simulink model "PassiveBalancingModelling"  (R2024b)
settings: Solver=FixedStepAuto  StartTime=0.0  StopTime=200  FixedStep=1e-3  RelTol=1e-3
model workspace (MAT data in the model file):
  Ah = 3
  R = 0.1
  SoC1 = 60
  SoC2 = 70
  SoC3 = 50
  SoC4 = 80
  Vnom = 3.7
undefined symbols (not defined in the file): Ion, Lithium
libraries: spsBatteryLib x4, spsIdealSwitchLib x4, spsSeriesRLCBranchLib x4, sps_lib x1
settings Model: Creator=MOHAMED  LastModifiedBy=MOHAMED

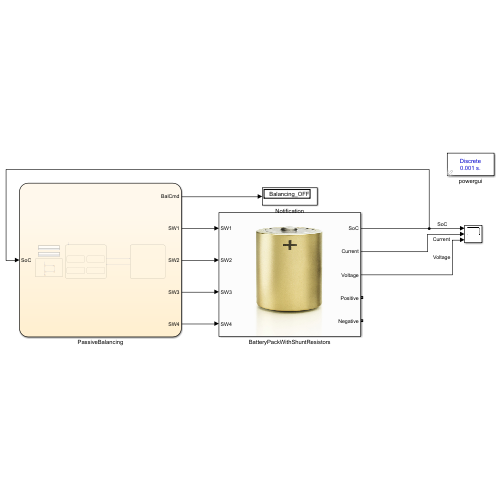
[thumbnail: Simulink's stored preview of the top-level diagram]
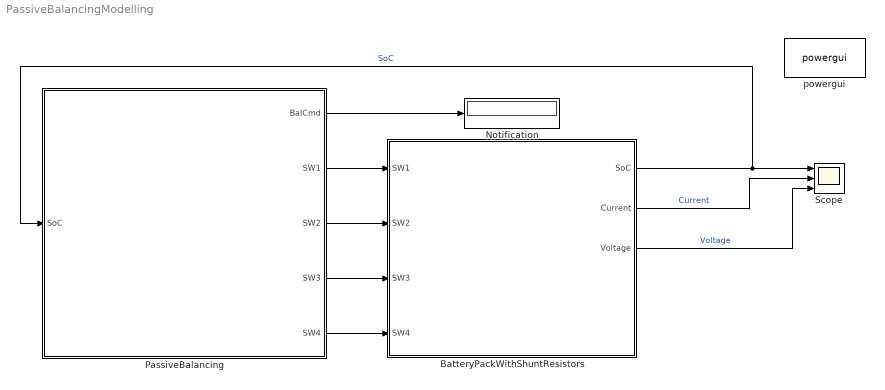
== system PassiveBalancingModelling ==
  BatteryPackWithShuntResistors : Subsystem
      mask Display: image('battery.jpg');
  Notification : Display
  PassiveBalancing : Stateflow chart  TreatAsAtomicUnit=on
  Scope : Scope  NumInputPorts=3
  powergui : sps_lib/powergui  Priority=1  SimulationMode=Discrete  SampleTime=1e-3  frequency=60  Iterations=50  frequencyindice=0  Pbase=100e6  ErrMax=1e-4  UnitsV=kV  UnitsW=MW  buscounter=0  FunctionMessages=off  echomessages=off  EnableUseOfTLC=off  CurrentSourceSwitches=off  DisableSnubberDevices=off  DisableRonSwitches=off  DisableVfSwitches=off  DisplayEquations=off  AutomaticDiscreteSolvers=off  SolverType=Tustin/Backward Euler (TBE)  Interpol=off  ExternalGateDelay=off  methode=off  Ts=100  x0status=blocks  SPID=on  SwTol=0  HookPort=off  NonlinearTolerance=1e-4  nMaxIteration=100  ContinueOnMaxIteration=off  RestoreLinks=warning  ResistiveCurrentMeasurement=off  Frange=[0:2:500]  Ylog=off  Xlog=on  ShowGrid=off  save=off  variable=ZData  structure=0  ZoomFFT=off  StartTime=0.0  cycles=1  DisplayStyle=1  fundamental=60  FreqAxis=off  MaxFrequency=1000  frequencyindicesteady=1  RmsSteady=1  display=off
  wires:
  BatteryPackWithShuntResistors/1(SoC) -> PassiveBalancing/1(SoC), Scope/1  "SoC"
  BatteryPackWithShuntResistors/2(Current) -> Scope/2  "Current"
  BatteryPackWithShuntResistors/3(Voltage) -> Scope/3  "Voltage"
  PassiveBalancing/1(BalCmd) -> Notification/1
  PassiveBalancing/2(SW1) -> BatteryPackWithShuntResistors/1(SW1)
  PassiveBalancing/3(SW2) -> BatteryPackWithShuntResistors/2(SW2)
  PassiveBalancing/4(SW3) -> BatteryPackWithShuntResistors/3(SW3)
  PassiveBalancing/5(SW4) -> BatteryPackWithShuntResistors/4(SW4)

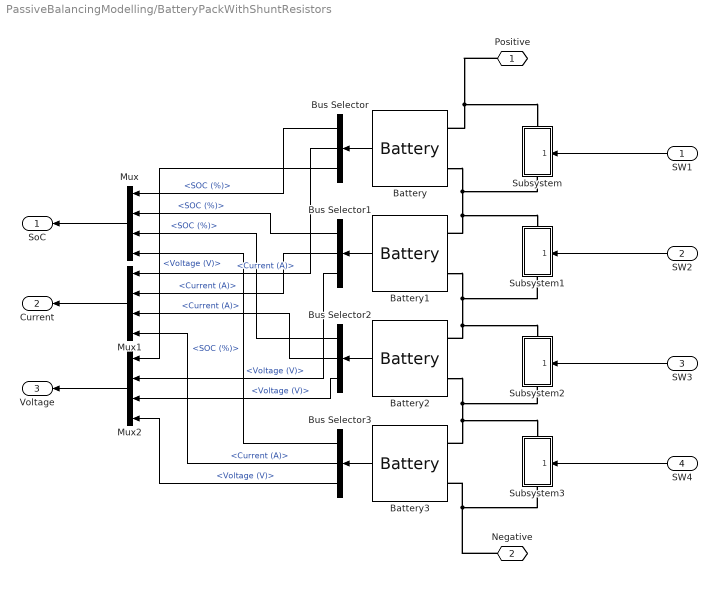
== system PassiveBalancingModelling/BatteryPackWithShuntResistors ==
  SW1 : Inport
  SW2 : Inport  Port=2
  SW3 : Inport  Port=3
  SW4 : Inport  Port=4
  Battery : spsBatteryLib/Battery  BatType=Lithium-Ion  NomV=Vnom  NomQ=Ah  SOC=SoC1  Batt_Tr=20e-3  PresetModel=on  MaxQ=3  MinV=2.775  FullV=4.3068  Dis_rate=1.3043  R=0.012333  Normal_OP=2.713  expZone="[3.9974     0.14739]"
  Battery1 : spsBatteryLib/Battery  BatType=Lithium-Ion  NomV=Vnom  NomQ=Ah  SOC=SoC2  Batt_Tr=20e-3  PresetModel=on  MaxQ=3  MinV=2.775  FullV=4.3068  Dis_rate=1.3043  R=0.012333  Normal_OP=2.713  expZone="[3.9974     0.14739]"
  Battery2 : spsBatteryLib/Battery  BatType=Lithium-Ion  NomV=Vnom  NomQ=Ah  SOC=SoC3  Batt_Tr=20e-3  PresetModel=on  MaxQ=3  MinV=2.775  FullV=4.3068  Dis_rate=1.3043  R=0.012333  Normal_OP=2.713  expZone="[3.9974     0.14739]"
  Battery3 : spsBatteryLib/Battery  BatType=Lithium-Ion  NomV=Vnom  NomQ=Ah  SOC=SoC4  Batt_Tr=20e-3  PresetModel=on  MaxQ=3  MinV=2.775  FullV=4.3068  Dis_rate=1.3043  R=0.012333  Normal_OP=2.713  expZone="[3.9974     0.14739]"
  Bus Selector{,1..3} (4 alike) : BusSelector  OutputSignals=SOC (%),Current (A),Voltage (V)
  Mux : Mux
  Mux1 : Mux
  Mux2 : Mux
  Subsystem : Subsystem
      settings: PortSchema="{\"entries\":[{\"content\":{\"sides\":[{\"content\":{\"connectorIds\":[\"LConn1\"]},\"type\":\"ConnectorPlacement.EquallySpacedRectSide\",\"uuid\":\"257d9981-230f-4391-a2c1-b56ae4b7ce10\"},{\"content\":{\"connectorIds\":[\"RConn1\"],\"side\":\"RIGHT\"},\"type\":\"ConnectorPlacement.EquallySpacedRectSide\",\"uuid\":\"90dd2fe2-2012-4c72-baa4-e13b85a759c3\"},{\"content\":{\"side\":\"TOP\"},\"type\":\"ConnectorPlacement.EquallySpacedRectSide\",\"uuid\":\"f37524ef-904f-4ff0-92c1-10d0565a33a2\"},{\"content\":{\"connectorIds\":[\"In1\"],\"side\":\"BOTTOM\"},\"type\":\"ConnectorPlacement.EquallySpacedRectSide\",\"uuid\":\"9c9ec85f-2592-4e7a-a4ab-a97d1a48809e\"}]},\"type\":\"ConnectorPlacement.EquallySpacedConnector\",\"uuid\":\"5659d0fe-4d8b-46d1-9b44-b48eced08a2e\"}],\"packageUris\":[\"http://schema.mathworks.com/mf0/Connector/R2020b\"],\"version\":\"1.0\"}"
  Subsystem1 : Subsystem
      settings: PortSchema="{\"entries\":[{\"content\":{\"sides\":[{\"content\":{\"connectorIds\":[\"LConn1\"]},\"type\":\"ConnectorPlacement.EquallySpacedRectSide\",\"uuid\":\"257d9981-230f-4391-a2c1-b56ae4b7ce10\"},{\"content\":{\"connectorIds\":[\"RConn1\"],\"side\":\"RIGHT\"},\"type\":\"ConnectorPlacement.EquallySpacedRectSide\",\"uuid\":\"90dd2fe2-2012-4c72-baa4-e13b85a759c3\"},{\"content\":{\"side\":\"TOP\"},\"type\":\"ConnectorPlacement.EquallySpacedRectSide\",\"uuid\":\"f37524ef-904f-4ff0-92c1-10d0565a33a2\"},{\"content\":{\"connectorIds\":[\"In1\"],\"side\":\"BOTTOM\"},\"type\":\"ConnectorPlacement.EquallySpacedRectSide\",\"uuid\":\"98333fe3-4431-4c4d-b596-c8152de66e7e\"}]},\"type\":\"ConnectorPlacement.EquallySpacedConnector\",\"uuid\":\"5659d0fe-4d8b-46d1-9b44-b48eced08a2e\"}],\"packageUris\":[\"http://schema.mathworks.com/mf0/Connector/R2020b\"],\"version\":\"1.0\"}"
  Subsystem2 : Subsystem
      settings: PortSchema="{\"entries\":[{\"content\":{\"sides\":[{\"content\":{\"connectorIds\":[\"LConn1\"]},\"type\":\"ConnectorPlacement.EquallySpacedRectSide\",\"uuid\":\"257d9981-230f-4391-a2c1-b56ae4b7ce10\"},{\"content\":{\"connectorIds\":[\"RConn1\"],\"side\":\"RIGHT\"},\"type\":\"ConnectorPlacement.EquallySpacedRectSide\",\"uuid\":\"90dd2fe2-2012-4c72-baa4-e13b85a759c3\"},{\"content\":{\"side\":\"TOP\"},\"type\":\"ConnectorPlacement.EquallySpacedRectSide\",\"uuid\":\"f37524ef-904f-4ff0-92c1-10d0565a33a2\"},{\"content\":{\"connectorIds\":[\"In1\"],\"side\":\"BOTTOM\"},\"type\":\"ConnectorPlacement.EquallySpacedRectSide\",\"uuid\":\"db011690-019c-4e6f-8d1a-cd9a411d2d3a\"}]},\"type\":\"ConnectorPlacement.EquallySpacedConnector\",\"uuid\":\"5659d0fe-4d8b-46d1-9b44-b48eced08a2e\"}],\"packageUris\":[\"http://schema.mathworks.com/mf0/Connector/R2020b\"],\"version\":\"1.0\"}"
  Subsystem3 : Subsystem
      settings: PortSchema="{\"entries\":[{\"content\":{\"sides\":[{\"content\":{\"connectorIds\":[\"LConn1\"]},\"type\":\"ConnectorPlacement.EquallySpacedRectSide\",\"uuid\":\"257d9981-230f-4391-a2c1-b56ae4b7ce10\"},{\"content\":{\"connectorIds\":[\"RConn1\"],\"side\":\"RIGHT\"},\"type\":\"ConnectorPlacement.EquallySpacedRectSide\",\"uuid\":\"90dd2fe2-2012-4c72-baa4-e13b85a759c3\"},{\"content\":{\"side\":\"TOP\"},\"type\":\"ConnectorPlacement.EquallySpacedRectSide\",\"uuid\":\"f37524ef-904f-4ff0-92c1-10d0565a33a2\"},{\"content\":{\"connectorIds\":[\"In1\"],\"side\":\"BOTTOM\"},\"type\":\"ConnectorPlacement.EquallySpacedRectSide\",\"uuid\":\"e69855d7-45e1-4b72-81ac-c9c0338e5721\"}]},\"type\":\"ConnectorPlacement.EquallySpacedConnector\",\"uuid\":\"5659d0fe-4d8b-46d1-9b44-b48eced08a2e\"}],\"packageUris\":[\"http://schema.mathworks.com/mf0/Connector/R2020b\"],\"version\":\"1.0\"}"
  Positive : PMIOPort  Side=Right
  Negative : PMIOPort  Port=2  Side=Right
  SoC : Outport
  Current : Outport  Port=2
  Voltage : Outport  Port=3
  wires:
  Mux1/1 -> Current/1
  Mux2/1 -> Voltage/1
  Mux/1 -> SoC/1
  Bus Selector3/3 -> Mux2/4  "<Voltage (V)>"
  Bus Selector2/3 -> Mux2/3  "<Voltage (V)>"
  Bus Selector/3 -> Mux2/1  "<Voltage (V)>"
  Bus Selector3/2 -> Mux1/4  "<Current (A)>"
  Bus Selector2/2 -> Mux1/3  "<Current (A)>"
  Bus Selector1/3 -> Mux2/2  "<Voltage (V)>"
  Bus Selector1/2 -> Mux1/2  "<Current (A)>"
  Bus Selector/2 -> Mux1/1  "<Current (A)>"
  Bus Selector3/1 -> Mux/4  "<SOC (%)>"
  Bus Selector2/1 -> Mux/3  "<SOC (%)>"
  Bus Selector1/1 -> Mux/2  "<SOC (%)>"
  Bus Selector/1 -> Mux/1  "<SOC (%)>"
  Battery2/1 -> Bus Selector2/1
  Battery3/1 -> Bus Selector3/1
  Battery1/1 -> Bus Selector1/1
  Battery/1 -> Bus Selector/1
  SW2/1 -> Subsystem1/1(SW2)
  SW3/1 -> Subsystem2/1(SW3)
  SW4/1 -> Subsystem3/1(SW4)
  SW1/1 -> Subsystem/1(SW1)
  connections:
  Negative/RConn1 -- Battery3/LConn2 -- Subsystem3/RConn1
  Positive/RConn1 -- Battery/LConn1 -- Subsystem/LConn1
  Battery2/LConn2 -- Subsystem2/RConn1 -- Subsystem3/LConn1 -- Battery3/LConn1
  Battery1/LConn2 -- Subsystem1/RConn1 -- Subsystem2/LConn1 -- Battery2/LConn1
  Battery/LConn2 -- Subsystem1/LConn1 -- Battery1/LConn1 -- Subsystem/RConn1

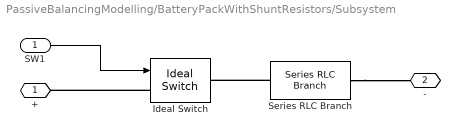
== system PassiveBalancingModelling/BatteryPackWithShuntResistors/Subsystem ==
  SW1 : Inport
  Ideal Switch : spsIdealSwitchLib/Ideal Switch  Ron=0.001  Lon=0  IC=0  Rs=1e5  Cs=inf  Measurements=off
  Series RLC Branch : spsSeriesRLCBranchLib/Series RLC Branch  LConnTagsString=__new0  RConnTagsString=__new0  BranchType=R  Resistance=R  Inductance=1e-3  SetiL0=off  InitialCurrent=0  Capacitance=1e-6  Setx0=off  InitialVoltage=0  Measurements=None
  + : PMIOPort  Side=Left
  - : PMIOPort  Port=2  Side=Right
  wires:
  SW1/1 -> Ideal Switch/1
  connections:
  Ideal Switch/LConn1 -- +/RConn1
  Series RLC Branch/LConn1 -- Ideal Switch/RConn1
  Series RLC Branch/RConn1 -- -/RConn1

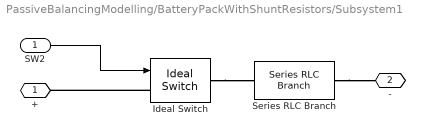
== system PassiveBalancingModelling/BatteryPackWithShuntResistors/Subsystem1 ==
  SW2 : Inport
  Ideal Switch : spsIdealSwitchLib/Ideal Switch  Ron=0.001  Lon=0  IC=0  Rs=1e5  Cs=inf  Measurements=off
  Series RLC Branch : spsSeriesRLCBranchLib/Series RLC Branch  LConnTagsString=__new0  RConnTagsString=__new0  BranchType=R  Resistance=R  Inductance=1e-3  SetiL0=off  InitialCurrent=0  Capacitance=1e-6  Setx0=off  InitialVoltage=0  Measurements=None
  + : PMIOPort  Side=Left
  - : PMIOPort  Port=2  Side=Right
  wires:
  SW2/1 -> Ideal Switch/1
  connections:
  Ideal Switch/RConn1 -- Series RLC Branch/LConn1
  Ideal Switch/LConn1 -- +/RConn1
  Series RLC Branch/RConn1 -- -/RConn1

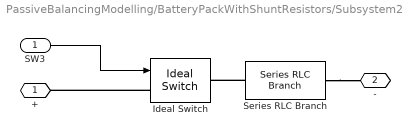
== system PassiveBalancingModelling/BatteryPackWithShuntResistors/Subsystem2 ==
  SW3 : Inport
  Ideal Switch : spsIdealSwitchLib/Ideal Switch  Ron=0.001  Lon=0  IC=0  Rs=1e5  Cs=inf  Measurements=off
  Series RLC Branch : spsSeriesRLCBranchLib/Series RLC Branch  LConnTagsString=__new0  RConnTagsString=__new0  BranchType=R  Resistance=R  Inductance=1e-3  SetiL0=off  InitialCurrent=0  Capacitance=1e-6  Setx0=off  InitialVoltage=0  Measurements=None
  + : PMIOPort  Side=Left
  - : PMIOPort  Port=2  Side=Right
  wires:
  SW3/1 -> Ideal Switch/1
  connections:
  Ideal Switch/LConn1 -- +/RConn1
  Series RLC Branch/LConn1 -- Ideal Switch/RConn1
  Series RLC Branch/RConn1 -- -/RConn1

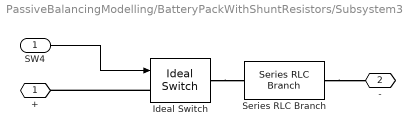
== system PassiveBalancingModelling/BatteryPackWithShuntResistors/Subsystem3 ==
  SW4 : Inport
  Ideal Switch : spsIdealSwitchLib/Ideal Switch  Ron=0.001  Lon=0  IC=0  Rs=1e5  Cs=inf  Measurements=off
  Series RLC Branch : spsSeriesRLCBranchLib/Series RLC Branch  LConnTagsString=__new0  RConnTagsString=__new0  BranchType=R  Resistance=R  Inductance=1e-3  SetiL0=off  InitialCurrent=0  Capacitance=1e-6  Setx0=off  InitialVoltage=0  Measurements=None
  + : PMIOPort  Side=Left
  - : PMIOPort  Port=2  Side=Right
  wires:
  SW4/1 -> Ideal Switch/1
  connections:
  Ideal Switch/LConn1 -- +/RConn1
  Ideal Switch/RConn1 -- Series RLC Branch/LConn1
  Series RLC Branch/RConn1 -- -/RConn1

== stateflow chart PassiveBalancingModelling/PassiveBalancing ==
  state BalancingON
    en, du:
    BalCmd = Command.Balancing_ON;
    Lowest = Min_SoC(SoC(1), SoC(2), SoC(3), SoC(4));
    state ControlSW1 [parallel]
      en, du:
      SW1 = ControlSW(SoC(1), Lowest);
      settings: executionOrder=1
    state ControlSW2 [parallel]
      en, du:
      SW2 = ControlSW(SoC(2), Lowest);
      settings: executionOrder=2
    state ControlSW3 [parallel]
      en, du:
      SW3 = ControlSW(SoC(3), Lowest);
      settings: executionOrder=3
    state ControlSW4 [parallel]
      en, du:
      SW4 = ControlSW(SoC(4), Lowest);
      settings: executionOrder=4
  state BalancingOFF
    en:
    BalCmd = Command.Balancing_OFF;
  state SW = ControlSW(SoC, Low) [function]
    (default) -> (junction 58) : % Switch Activation
    (junction 58) -> (junction 59) [order 1] : [abs(SoC - Low) > 0.01]
    (junction 58) -> (junction 60) [order 2] : {SW = 0;}
    (junction 59) -> (junction 61) : {SW = 1;}
    (junction 61) -> (junction 60)
    (junction 60) -> (junction 62)
  (default) -> BalancingON
  BalancingON -> BalancingOFF : [BalOFF(SoC(1), SoC(2), SoC(3), SoC(4))]
  BalancingOFF -> BalancingON : [~BalOFF(SoC(1), SoC(2), SoC(3), SoC(4))]
  data: SoC1 function_input double; SoC2 function_input double; SoC3 function_input double; SoC4 function_input double; out function_output double; SoC1 function_input double; SoC2 function_input double; SoC3 function_input double; SoC4 function_input double; out function_output double; SoC function_input; SW function_output; Low function_input; BalCmd output; SoC input; SW1 output; SW2 output; SW3 output; SW4 output; Lowest local
  function out = Min_SoC(SoC1, SoC2, SoC3, SoC4):
    | function out = Min_SoC(SoC1, SoC2, SoC3, SoC4)
    |     out = min(SoC1, min(SoC2, min(SoC3, SoC4)));
    | end
  function out = BalOFF(SoC1, SoC2, SoC3, SoC4):
    | function out = BalOFF(SoC1, SoC2, SoC3, SoC4)
    |     if(abs(SoC1 - SoC2) > 0.001 && abs(SoC1 - SoC3) > 0.001 && abs(SoC1 - SoC4) > 0.001)
    |         out = 1;
    |     else
    |         out = 0;
    |     end
    | end
